simulink model "m_ary_BPSK_10240"  (R2021b)
settings: Solver=VariableStepAuto  StartTime=0.0  StopTime=0.001250  RelTol=1e-3
libraries: dsparch4 x4, commfilt2 x4, commchan3 x1, commrandsrc3 x1
settings Model: Creator=Sujay  LastModifiedBy=Sujay

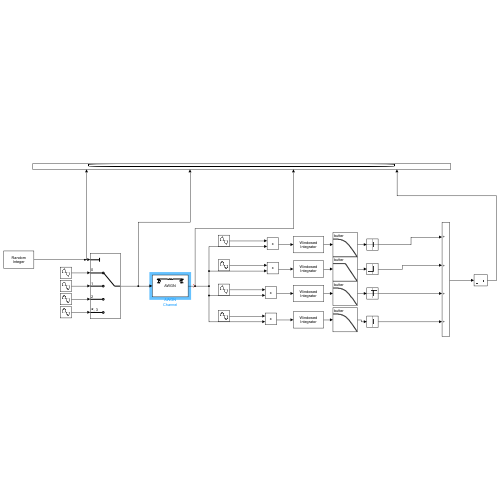
[thumbnail: Simulink's stored preview of the top-level diagram]
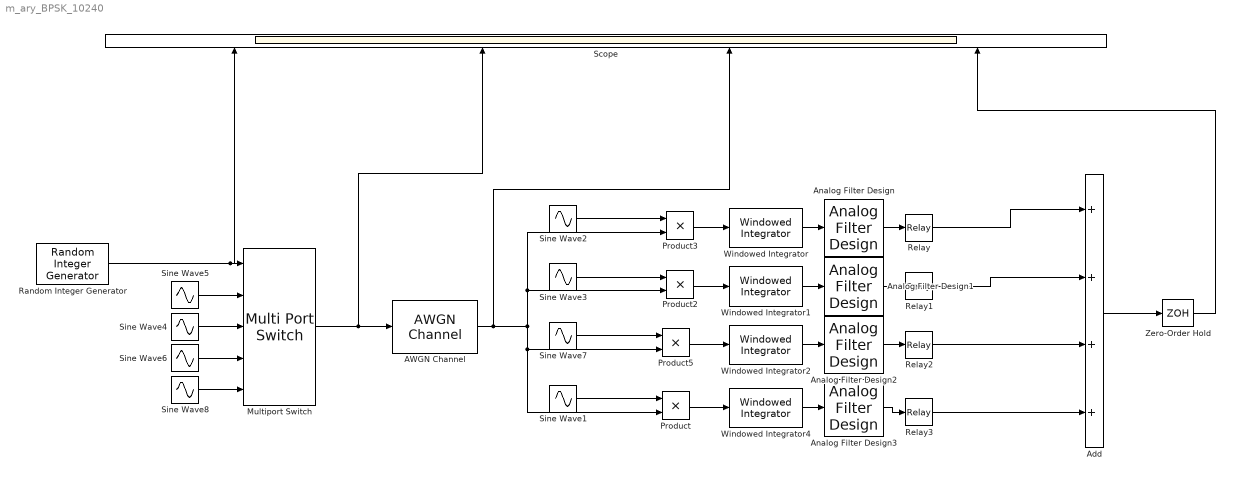
== system m_ary_BPSK_10240 ==
  AWGN Channel : commchan3/AWGN Channel  InputProcessing=Columns as channels (frame based)  seed=67  noiseMode="Signal to noise ratio  (SNR)"  EbNodB=10  EsNodB=10  SNRdB=20  bitsPerSym=1  Ps=1  Tsym=1  variance=1
  Add : Sum  Inputs=++++
  Analog Filter Design : dsparch4/Analog Filter Design  method=Butterworth  filttype=Lowpass  N=1  Wlo=2 * pi * 24 * 1000  Whi=80  Rp=2  Rs=40
  Analog Filter Design1 : dsparch4/Analog Filter Design  method=Butterworth  filttype=Lowpass  N=8  Wlo=2*pi*24*1000  Whi=80  Rp=2  Rs=40
  Analog Filter Design2 : dsparch4/Analog Filter Design  method=Butterworth  filttype=Lowpass  N=1  Wlo=2*pi*24*1000  Whi=80  Rp=2  Rs=40
  Analog Filter Design3 : dsparch4/Analog Filter Design  method=Butterworth  filttype=Lowpass  N=1  Wlo=2*pi*24*1000  Whi=80  Rp=2  Rs=40
  Multiport Switch : MultiPortSwitch  DataPortOrder=Zero-based contiguous  Inputs=4  zeroidx=on
  Product{,2..3,5} (4 alike) : Product
  Random Integer Generator : commrandsrc3/Random Integer Generator  SetSize=4  SeedSource=Auto  Seed=0  SampleTime=1/10240  SamplesPerFrame=1  OutputDataType=double  SimulateUsing=Interpreted execution
  Relay : Relay  OnSwitchValue=15  OffSwitchValue=5  OnOutputValue=0
  Relay1 : Relay  OnSwitchValue=15  OffSwitchValue=5
  Relay2 : Relay  OnSwitchValue=15  OffSwitchValue=5  OnOutputValue=2
  Relay3 : Relay  OnSwitchValue=15  OffSwitchValue=5  OnOutputValue=3
  Scope : Scope  NumInputPorts=4
  Sine Wave1 : Sin  Frequency=2 * pi * 24 * 1000  Phase=3 * pi /2  SampleTime=0.000001
  Sine Wave2 : Sin  Frequency=2 * pi * 24 * 1000  SampleTime=0.000001
  Sine Wave3 : Sin  Frequency=2 * pi * 24 * 1000  Phase=pi/2  SampleTime=0.000001
  Sine Wave4 : Sin  Frequency=2 * pi * 24 * 1000  Phase=pi/2  SampleTime=0.000001
  Sine Wave5 : Sin  Frequency=2 * pi * 24 * 1000  SampleTime=0.000001
  Sine Wave6 : Sin  Frequency=2 * pi * 24 * 1000  Phase=pi  SampleTime=0.000001
  Sine Wave7 : Sin  Frequency=2 * pi * 24 * 1000  Phase=pi  SampleTime=0.000001
  Sine Wave8 : Sin  Frequency=2 * pi * 24 * 1000  Phase=3 * pi /2  SampleTime=0.000001
  Windowed Integrator{,1..2,4} (4 alike) : commfilt2/Windowed Integrator  integperiod=42  InputProcessing=Columns as channels (frame based)  roundingMode=Floor  overflowMode=off  coeffDataTypeStr=Inherit: Same word length as input  coeffMin=[]  coeffMax=[]  coeffLastDataTypeStr=Inherit: Same word length as input  accumDataTypeStr=Inherit: Same as product output  accumLastDataTypeStr=Inherit: Same as product output  outputDataTypeStr=Inherit: Same as accumulator  outputMin=[]  outputMax=[]  outputLastDataTypeStr=Inherit: Same as accumulator
      settings: SourceProductBaseCode=CM
  Zero-Order Hold : ZeroOrderHold  SampleTime=1/10240
  wires:
  Sine Wave3/1 -> Product2/1
  Sine Wave2/1 -> Product3/1
  Product3/1 -> Windowed Integrator/1
  Product2/1 -> Windowed Integrator1/1
  Random Integer Generator/1 -> Scope/1, Multiport Switch/1
  Sine Wave5/1 -> Multiport Switch/2
  Sine Wave4/1 -> Multiport Switch/3
  Sine Wave6/1 -> Multiport Switch/4
  Sine Wave8/1 -> Multiport Switch/5
  Multiport Switch/1 -> Scope/2, AWGN Channel/1
  Sine Wave7/1 -> Product5/1
  Product5/1 -> Windowed Integrator2/1
  AWGN Channel/1 -> Scope/3, Product2/2, Product3/2, Product/2, Product5/2
  Product/1 -> Windowed Integrator4/1
  Sine Wave1/1 -> Product/1
  Windowed Integrator/1 -> Analog Filter Design/1
  Windowed Integrator1/1 -> Analog Filter Design1/1
  Windowed Integrator2/1 -> Analog Filter Design2/1
  Relay/1 -> Add/1
  Relay1/1 -> Add/2
  Relay2/1 -> Add/3
  Relay3/1 -> Add/4
  Add/1 -> Zero-Order Hold/1
  Analog Filter Design/1 -> Relay/1
  Analog Filter Design1/1 -> Relay1/1
  Analog Filter Design2/1 -> Relay2/1
  Windowed Integrator4/1 -> Analog Filter Design3/1
  Analog Filter Design3/1 -> Relay3/1
  Zero-Order Hold/1 -> Scope/4
